simulink model "PX4_Run_Mode_R2016b"  (R2017b)
settings: Solver=FixedStepDiscrete  StartTime=0.0  StopTime=inf  FixedStep=Ts  RelTol=1e-3  EnableMultiTasking=on
InitFcn:
  | run('InitFcn_R2016b.m');
values from neighbouring files (symbols this model uses):
  A = Pixhawk_CSC.Parameter( {single([diag([1 1 1]) Ts*diag([1 1 1]); diag([0 0 0]) diag([1 1 1])]),'A'} )    [InitFcn.m]    (also in InitFcn_R2016b.m; InitFcn_R2017b_no_csc.m = single([diag([1 1 1]) Ts*diag([1 1 1]); diag([0 0 0]) diag([)
  app = Pixhawk_CSC.Parameter({single( [0.05; 0.05; 0.05]),'app'} )    [InitFcn.m]    (also in InitFcn_R2016b.m; InitFcn_R2017b_no_csc.m = single( [0.05; 0.05; 0.05]))
  B = Pixhawk_CSC.Parameter( {single([Ts^2/2*diag([1 1 1]); Ts*diag([1 1 1])]),'B'} )    [InitFcn.m]    (also in InitFcn_R2016b.m; InitFcn_R2017b_no_csc.m = single([Ts^2/2*diag([1 1 1]); Ts*diag([1 1 1])]))
  Beta = Pixhawk_CSC.Parameter({single( 0.02),'Beta'} )    [InitFcn.m]    (also in InitFcn_R2016b.m; InitFcn_R2017b_no_csc.m = single( 0.02))
  C = Pixhawk_CSC.Parameter( {single([diag([1 1 1]) 0*diag([1 1 1]); zeros(1,2) 1 zeros(1,3)]),'C'} )    [InitFcn.m]    (also in InitFcn_R2016b.m; InitFcn_R2017b_no_csc.m = single([diag([1 1 1]) 0*diag([1 1 1]); zeros(1,2) 1 zeros(1,)
  C1 = Pixhawk_CSC.Parameter({single( 1.08680),'C1'} )    [InitFcn.m]    (also in InitFcn_R2016b.m; InitFcn_R2017b_no_csc.m = single( 1.08680))
  C10 = Pixhawk_CSC.Parameter({single( 0.0000),'C10'} )    [InitFcn.m]    (also in InitFcn_R2016b.m; InitFcn_R2017b_no_csc.m = single( 0.0000))
  C11 = Pixhawk_CSC.Parameter({single(-0.2300),'C11'} )    [InitFcn.m]    (also in InitFcn_R2016b.m; InitFcn_R2017b_no_csc.m = single(-0.2300))
  C12 = Pixhawk_CSC.Parameter({single( 0.0000),'C12'} )    [InitFcn.m]    (also in InitFcn_R2016b.m; InitFcn_R2017b_no_csc.m = single( 0.0000))
  C13 = Pixhawk_CSC.Parameter({single( 0.8000),'C13'} )    [InitFcn.m]    (also in InitFcn_R2016b.m; InitFcn_R2017b_no_csc.m = single( 0.8000))
  C14 = Pixhawk_CSC.Parameter({single( 0.8000),'C14'} )    [InitFcn.m]    (also in InitFcn_R2016b.m; InitFcn_R2017b_no_csc.m = single( 0.8000))
  C15 = Pixhawk_CSC.Parameter({single( 1.73200),'C15'} )    [InitFcn.m]    (also in InitFcn_R2016b.m; InitFcn_R2017b_no_csc.m = single( 1.73200))
  C16 = Pixhawk_CSC.Parameter({single( 0.1000),'C16'} )    [InitFcn.m]    (also in InitFcn_R2016b.m; InitFcn_R2017b_no_csc.m = single( 0.1000))
  C17 = Pixhawk_CSC.Parameter({single( 0.1000),'C17'} )    [InitFcn.m]    (also in InitFcn_R2016b.m; InitFcn_R2017b_no_csc.m = single( 0.1000))
  C18 = Pixhawk_CSC.Parameter({single( 0.0500),'C18'} )    [InitFcn.m]    (also in InitFcn_R2016b.m; InitFcn_R2017b_no_csc.m = single( 0.0500))
  C19 = Pixhawk_CSC.Parameter({single( 0.6000),'C19'} )    [InitFcn.m]    (also in InitFcn_R2016b.m; InitFcn_R2017b_no_csc.m = single( 0.6000))
  C2 = Pixhawk_CSC.Parameter({single( 1.10468),'C2'} )    [InitFcn.m]    (also in InitFcn_R2016b.m; InitFcn_R2017b_no_csc.m = single( 1.10468))
  C20 = Pixhawk_CSC.Parameter({single( 0.6000),'C20'} )    [InitFcn.m]    (also in InitFcn_R2016b.m; InitFcn_R2017b_no_csc.m = single( 0.6000))
  C21 = Pixhawk_CSC.Parameter({single( 1.04558),'C21'} )    [InitFcn.m]    (also in InitFcn_R2016b.m; InitFcn_R2017b_no_csc.m = single( 1.04558))
  C22 = Pixhawk_CSC.Parameter({single( 0.0000),'C22'} )    [InitFcn.m]    (also in InitFcn_R2016b.m; InitFcn_R2017b_no_csc.m = single( 0.0000))
  C23 = Pixhawk_CSC.Parameter({single( 0.0000),'C23'} )    [InitFcn.m]    (also in InitFcn_R2016b.m; InitFcn_R2017b_no_csc.m = single( 0.0000))
  C24 = Pixhawk_CSC.Parameter({single(-11.0000),'C24'} )    [InitFcn.m]    (also in InitFcn_R2016b.m; InitFcn_R2017b_no_csc.m = single(-11.0000))
  C3 = Pixhawk_CSC.Parameter({single( 1.1980),'C3'} )    [InitFcn.m]    (also in InitFcn_R2016b.m; InitFcn_R2017b_no_csc.m = single( 1.1980))
  C4 = Pixhawk_CSC.Parameter({single( 0.0500),'C4'} )    [InitFcn.m]    (also in InitFcn_R2016b.m; InitFcn_R2017b_no_csc.m = single( 0.0500))
  C5 = Pixhawk_CSC.Parameter({single( 0.0500),'C5'} )    [InitFcn.m]    (also in InitFcn_R2016b.m; InitFcn_R2017b_no_csc.m = single( 0.0500))
  C6 = Pixhawk_CSC.Parameter({single( 0.0500),'C6'} )    [InitFcn.m]    (also in InitFcn_R2016b.m; InitFcn_R2017b_no_csc.m = single( 0.0500))
  C7 = Pixhawk_CSC.Parameter({single( 0.35937),'C7'} )    [InitFcn.m]    (also in InitFcn_R2016b.m; InitFcn_R2017b_no_csc.m = single( 0.35937))
  C8 = Pixhawk_CSC.Parameter({single( 0.36528),'C8'} )    [InitFcn.m]    (also in InitFcn_R2016b.m; InitFcn_R2017b_no_csc.m = single( 0.36528))
  C9 = Pixhawk_CSC.Parameter({single( 0.53311),'C9'} )    [InitFcn.m]    (also in InitFcn_R2016b.m; InitFcn_R2017b_no_csc.m = single( 0.53311))
  C_1 = Pixhawk_CSC.Parameter( {single([diag([1 1 1]) 0*diag([1 1 1])]),'C1'} )    [InitFcn.m]    (also in InitFcn_R2016b.m; InitFcn_R2017b_no_csc.m = single([diag([1 1 1]) 0*diag([1 1 1])]))
  CAL_ACC0_XOFFSET = Pixhawk_CSC.Parameter( {single( 0.122052  ),'CAL_ACC0_XOFFSET'} )    [InitFcn.m]    (also in InitFcn_R2016b.m; InitFcn_R2017b_no_csc.m = single( 0.122052  ))
  CAL_ACC0_XXSCALE = Pixhawk_CSC.Parameter( {single(  1.01218    ),'CAL_ACC0_XXSCALE'} )    [InitFcn.m]    (also in InitFcn_R2016b.m; InitFcn_R2017b_no_csc.m = single(  1.01218    ))
  CAL_ACC0_XYSCALE = Pixhawk_CSC.Parameter( {single( -0.00443301 ),'CAL_ACC0_XYSCALE'} )    [InitFcn.m]    (also in InitFcn_R2016b.m; InitFcn_R2017b_no_csc.m = single( -0.00443301 ))
  CAL_ACC0_XZSCALE = Pixhawk_CSC.Parameter( {single( -0.00505793 ),'CAL_ACC0_XZSCALE'} )    [InitFcn.m]    (also in InitFcn_R2016b.m; InitFcn_R2017b_no_csc.m = single( -0.00505793 ))
  CAL_ACC0_YOFFSET = Pixhawk_CSC.Parameter( {single( 0.00281205),'CAL_ACC0_YOFFSET'} )    [InitFcn.m]    (also in InitFcn_R2016b.m; InitFcn_R2017b_no_csc.m = single( 0.00281205))
  CAL_ACC0_YXSCALE = Pixhawk_CSC.Parameter( {single( -0.00443301 ),'CAL_ACC0_YXSCALE'} )    [InitFcn.m]    (also in InitFcn_R2016b.m; InitFcn_R2017b_no_csc.m = single( -0.00443301 ))
  CAL_ACC0_YYSCALE = Pixhawk_CSC.Parameter( {single(  1.00234    ),'CAL_ACC0_YYSCALE'} )    [InitFcn.m]    (also in InitFcn_R2016b.m; InitFcn_R2017b_no_csc.m = single(  1.00234    ))
  CAL_ACC0_YZSCALE = Pixhawk_CSC.Parameter( {single(  0.0160883  ),'CAL_ACC0_YZSCALE'} )    [InitFcn.m]    (also in InitFcn_R2016b.m; InitFcn_R2017b_no_csc.m = single(  0.0160883  ))
  CAL_ACC0_ZOFFSET = Pixhawk_CSC.Parameter( {single(-0.0298121 ),'CAL_ACC0_ZOFFSET'} )    [InitFcn.m]    (also in InitFcn_R2016b.m; InitFcn_R2017b_no_csc.m = single(-0.0298121 ))
  CAL_ACC0_ZXSCALE = Pixhawk_CSC.Parameter( {single( -0.00505793 ),'CAL_ACC0_ZXSCALE'} )    [InitFcn.m]    (also in InitFcn_R2016b.m; InitFcn_R2017b_no_csc.m = single( -0.00505793 ))
  CAL_ACC0_ZYSCALE = Pixhawk_CSC.Parameter( {single(  0.0160883  ),'CAL_ACC0_ZYSCALE'} )    [InitFcn.m]    (also in InitFcn_R2016b.m; InitFcn_R2017b_no_csc.m = single(  0.0160883  ))
  CAL_ACC0_ZZSCALE = Pixhawk_CSC.Parameter( {single(  0.983604   ),'CAL_ACC0_ZZSCALE'} )    [InitFcn.m]    (also in InitFcn_R2016b.m; InitFcn_R2017b_no_csc.m = single(  0.983604   ))
  CAL_BAR_OFFSET = Pixhawk_CSC.Parameter( {single( -20.8468),'CAL_BAR_OFFSET'} )    [InitFcn.m]    (also in InitFcn_R2016b.m; InitFcn_R2017b_no_csc.m = single( -20.8468))
  CAL_BAR_SCALE = Pixhawk_CSC.Parameter( {single(   1.0632),'CAL_BAR_SCALE'} )    [InitFcn.m]    (also in InitFcn_R2016b.m; InitFcn_R2017b_no_csc.m = single(   1.0632))
  CAL_BAT0_XOFFSET = Pixhawk_CSC.Parameter( {single( 0.0000),'CAL_BAT0_XOFFSET'} )    [InitFcn.m]    (also in InitFcn_R2016b.m; InitFcn_R2017b_no_csc.m = single( 0.0000))
  CAL_BAT0_XXSCALE = Pixhawk_CSC.Parameter( {single(  1.0000),'CAL_BAT0_XXSCALE'} )    [InitFcn.m]    (also in InitFcn_R2016b.m; InitFcn_R2017b_no_csc.m = single(  1.0000))
  CAL_BAT0_XYSCALE = Pixhawk_CSC.Parameter( {single(  0.0000),'CAL_BAT0_XYSCALE'} )    [InitFcn.m]    (also in InitFcn_R2016b.m; InitFcn_R2017b_no_csc.m = single(  0.0000))
  CAL_BAT0_XZSCALE = Pixhawk_CSC.Parameter( {single(  0.0000),'CAL_BAT0_XZSCALE'} )    [InitFcn.m]    (also in InitFcn_R2016b.m; InitFcn_R2017b_no_csc.m = single(  0.0000))
  CAL_BAT0_YOFFSET = Pixhawk_CSC.Parameter( {single( 0.0000),'CAL_BAT0_YOFFSET'} )    [InitFcn.m]    (also in InitFcn_R2016b.m; InitFcn_R2017b_no_csc.m = single( 0.0000))
  CAL_BAT0_YXSCALE = Pixhawk_CSC.Parameter( {single(  0.0000),'CAL_BAT0_YXSCALE'} )    [InitFcn.m]    (also in InitFcn_R2016b.m; InitFcn_R2017b_no_csc.m = single(  0.0000))
  CAL_BAT0_YYSCALE = Pixhawk_CSC.Parameter( {single(  1.0000),'CAL_BAT0_YYSCALE'} )    [InitFcn.m]    (also in InitFcn_R2016b.m; InitFcn_R2017b_no_csc.m = single(  1.0000))
  CAL_BAT0_YZSCALE = Pixhawk_CSC.Parameter( {single(  0.0000),'CAL_BAT0_YZSCALE'} )    [InitFcn.m]    (also in InitFcn_R2016b.m; InitFcn_R2017b_no_csc.m = single(  0.0000))
  CAL_BAT0_ZOFFSET = Pixhawk_CSC.Parameter( {single( 0.0000),'CAL_BAT0_ZOFFSET'} )    [InitFcn.m]    (also in InitFcn_R2016b.m; InitFcn_R2017b_no_csc.m = single( 0.0000))
  CAL_BAT0_ZXSCALE = Pixhawk_CSC.Parameter( {single(  0.0000),'CAL_BAT0_ZXSCALE'} )    [InitFcn.m]    (also in InitFcn_R2016b.m; InitFcn_R2017b_no_csc.m = single(  0.0000))
  CAL_BAT0_ZYSCALE = Pixhawk_CSC.Parameter( {single(  0.0000),'CAL_BAT0_ZYSCALE'} )    [InitFcn.m]    (also in InitFcn_R2016b.m; InitFcn_R2017b_no_csc.m = single(  0.0000))
  CAL_BAT0_ZZSCALE = Pixhawk_CSC.Parameter( {single(  1.0000),'CAL_BAT0_ZZSCALE'} )    [InitFcn.m]    (also in InitFcn_R2016b.m; InitFcn_R2017b_no_csc.m = single(  1.0000))
  CAL_GPS0_XOFFSET = Pixhawk_CSC.Parameter( {single( 0.0000),'CAL_GPS0_XOFFSET'} )    [InitFcn.m]    (also in InitFcn_R2016b.m; InitFcn_R2017b_no_csc.m = single( 0.0000))
  CAL_GPS0_XXSCALE = Pixhawk_CSC.Parameter( {single(  0.0100),'CAL_GPS0_XXSCALE'} )    [InitFcn.m]    (also in InitFcn_R2016b.m; InitFcn_R2017b_no_csc.m = single(  0.0100))
  CAL_GPS0_XYSCALE = Pixhawk_CSC.Parameter( {single(  0.0000),'CAL_GPS0_XYSCALE'} )    [InitFcn.m]    (also in InitFcn_R2016b.m; InitFcn_R2017b_no_csc.m = single(  0.0000))
  CAL_GPS0_XZSCALE = Pixhawk_CSC.Parameter( {single(  0.0000),'CAL_GPS0_XZSCALE'} )    [InitFcn.m]    (also in InitFcn_R2016b.m; InitFcn_R2017b_no_csc.m = single(  0.0000))
  CAL_GPS0_YOFFSET = Pixhawk_CSC.Parameter( {single( 0.0000),'CAL_GPS0_YOFFSET'} )    [InitFcn.m]    (also in InitFcn_R2016b.m; InitFcn_R2017b_no_csc.m = single( 0.0000))
  CAL_GPS0_YXSCALE = Pixhawk_CSC.Parameter( {single(  0.0000),'CAL_GPS0_YXSCALE'} )    [InitFcn.m]    (also in InitFcn_R2016b.m; InitFcn_R2017b_no_csc.m = single(  0.0000))
  CAL_GPS0_YYSCALE = Pixhawk_CSC.Parameter( {single(  0.0100),'CAL_GPS0_YYSCALE'} )    [InitFcn.m]    (also in InitFcn_R2016b.m; InitFcn_R2017b_no_csc.m = single(  0.0100))
  CAL_GPS0_YZSCALE = Pixhawk_CSC.Parameter( {single(  0.0000),'CAL_GPS0_YZSCALE'} )    [InitFcn.m]    (also in InitFcn_R2016b.m; InitFcn_R2017b_no_csc.m = single(  0.0000))
  CAL_GPS0_ZOFFSET = Pixhawk_CSC.Parameter( {single( 0.0000),'CAL_GPS0_ZOFFSET'} )    [InitFcn.m]    (also in InitFcn_R2016b.m; InitFcn_R2017b_no_csc.m = single( 0.0000))
  CAL_GPS0_ZXSCALE = Pixhawk_CSC.Parameter( {single(  0.0000),'CAL_GPS0_ZXSCALE'} )    [InitFcn.m]    (also in InitFcn_R2016b.m; InitFcn_R2017b_no_csc.m = single(  0.0000))
  CAL_GPS0_ZYSCALE = Pixhawk_CSC.Parameter( {single(  0.0000),'CAL_GPS0_ZYSCALE'} )    [InitFcn.m]    (also in InitFcn_R2016b.m; InitFcn_R2017b_no_csc.m = single(  0.0000))
  CAL_GPS0_ZZSCALE = Pixhawk_CSC.Parameter( {single( -0.0010),'CAL_GPS0_ZZSCALE'} )    [InitFcn.m]    (also in InitFcn_R2016b.m; InitFcn_R2017b_no_csc.m = single( -0.0010))
  CAL_GYRO0_XXSCALE = Pixhawk_CSC.Parameter( {single(0.992736),'CAL_GYRO0_XXSCALE'} )    [InitFcn.m]    (also in InitFcn_R2016b.m; InitFcn_R2017b_no_csc.m = single(0.992736))
  CAL_GYRO0_XYSCALE = Pixhawk_CSC.Parameter( {single(0.0000),'CAL_GYRO0_XYSCALE'} )    [InitFcn.m]    (also in InitFcn_R2016b.m; InitFcn_R2017b_no_csc.m = single(0.0000))
  CAL_GYRO0_XZSCALE = Pixhawk_CSC.Parameter( {single(0.0000),'CAL_GYRO0_XZSCALE'} )    [InitFcn.m]    (also in InitFcn_R2016b.m; InitFcn_R2017b_no_csc.m = single(0.0000))
  CAL_GYRO0_YXSCALE = Pixhawk_CSC.Parameter( {single(0.0000),'CAL_GYRO0_YXSCALE'} )    [InitFcn.m]    (also in InitFcn_R2016b.m; InitFcn_R2017b_no_csc.m = single(0.0000))
  CAL_GYRO0_YYSCALE = Pixhawk_CSC.Parameter( {single(1.01609),'CAL_GYRO0_YYSCALE'} )    [InitFcn.m]    (also in InitFcn_R2016b.m; InitFcn_R2017b_no_csc.m = single(1.01609))
  CAL_GYRO0_YZSCALE = Pixhawk_CSC.Parameter( {single(0.0000),'CAL_GYRO0_YZSCALE'} )    [InitFcn.m]    (also in InitFcn_R2016b.m; InitFcn_R2017b_no_csc.m = single(0.0000))
  CAL_GYRO0_ZXSCALE = Pixhawk_CSC.Parameter( {single(0.0000),'CAL_GYRO0_ZXSCALE'} )    [InitFcn.m]    (also in InitFcn_R2016b.m; InitFcn_R2017b_no_csc.m = single(0.0000))
  CAL_GYRO0_ZYSCALE = Pixhawk_CSC.Parameter( {single(0.0000),'CAL_GYRO0_ZYSCALE'} )    [InitFcn.m]    (also in InitFcn_R2016b.m; InitFcn_R2017b_no_csc.m = single(0.0000))
  CAL_GYRO0_ZZSCALE = Pixhawk_CSC.Parameter( {single(1.03003),'CAL_GYRO0_ZZSCALE'} )    [InitFcn.m]    (also in InitFcn_R2016b.m; InitFcn_R2017b_no_csc.m = single(1.03003))
  CAL_MAG0_XCURCOR = Pixhawk_CSC.Parameter( {single( 0.0017     ),'CAL_MAG0_XCURCOR'} )    [InitFcn.m]    (also in InitFcn_R2016b.m; InitFcn_R2017b_no_csc.m = single( 0.0017     ))
  CAL_MAG0_XOFFSET = Pixhawk_CSC.Parameter( {single( 0.0446372  ),'CAL_MAG0_XOFFSET'} )    [InitFcn.m]    (also in InitFcn_R2016b.m; InitFcn_R2017b_no_csc.m = single( 0.0446372  ))
  CAL_MAG0_XXSCALE = Pixhawk_CSC.Parameter( {single(  1.01563   ),'CAL_MAG0_XXSCALE'} )    [InitFcn.m]    (also in InitFcn_R2016b.m; InitFcn_R2017b_no_csc.m = single(  1.01563   ))
  CAL_MAG0_XYSCALE = Pixhawk_CSC.Parameter( {single( -0.0612061 ),'CAL_MAG0_XYSCALE'} )    [InitFcn.m]    (also in InitFcn_R2016b.m; InitFcn_R2017b_no_csc.m = single( -0.0612061 ))
  CAL_MAG0_XZSCALE = Pixhawk_CSC.Parameter( {single( -0.011532  ),'CAL_MAG0_XZSCALE'} )    [InitFcn.m]    (also in InitFcn_R2016b.m; InitFcn_R2017b_no_csc.m = single( -0.011532  ))
  CAL_MAG0_YCURCOR = Pixhawk_CSC.Parameter( {single(-0.0075     ),'CAL_MAG0_YCURCOR'} )    [InitFcn.m]    (also in InitFcn_R2016b.m; InitFcn_R2017b_no_csc.m = single(-0.0075     ))
  CAL_MAG0_YOFFSET = Pixhawk_CSC.Parameter( {single( 0.0700776  ),'CAL_MAG0_YOFFSET'} )    [InitFcn.m]    (also in InitFcn_R2016b.m; InitFcn_R2017b_no_csc.m = single( 0.0700776  ))
  CAL_MAG0_YXSCALE = Pixhawk_CSC.Parameter( {single( -0.0612061 ),'CAL_MAG0_YXSCALE'} )    [InitFcn.m]    (also in InitFcn_R2016b.m; InitFcn_R2017b_no_csc.m = single( -0.0612061 ))
  CAL_MAG0_YYSCALE = Pixhawk_CSC.Parameter( {single(  1.00593   ),'CAL_MAG0_YYSCALE'} )    [InitFcn.m]    (also in InitFcn_R2016b.m; InitFcn_R2017b_no_csc.m = single(  1.00593   ))
  CAL_MAG0_YZSCALE = Pixhawk_CSC.Parameter( {single(  0.0144582 ),'CAL_MAG0_YZSCALE'} )    [InitFcn.m]    (also in InitFcn_R2016b.m; InitFcn_R2017b_no_csc.m = single(  0.0144582 ))
  CAL_MAG0_ZCURCOR = Pixhawk_CSC.Parameter( {single(-0.0080     ),'CAL_MAG0_ZCURCOR'} )    [InitFcn.m]    (also in InitFcn_R2016b.m; InitFcn_R2017b_no_csc.m = single(-0.0080     ))
  CAL_MAG0_ZOFFSET = Pixhawk_CSC.Parameter( {single( 0.00201742 ),'CAL_MAG0_ZOFFSET'} )    [InitFcn.m]    (also in InitFcn_R2016b.m; InitFcn_R2017b_no_csc.m = single( 0.00201742 ))
  CAL_MAG0_ZXSCALE = Pixhawk_CSC.Parameter( {single( -0.011532  ),'CAL_MAG0_ZXSCALE'} )    [InitFcn.m]    (also in InitFcn_R2016b.m; InitFcn_R2017b_no_csc.m = single( -0.011532  ))
  CAL_MAG0_ZYSCALE = Pixhawk_CSC.Parameter( {single(  0.0144582 ),'CAL_MAG0_ZYSCALE'} )    [InitFcn.m]    (also in InitFcn_R2016b.m; InitFcn_R2017b_no_csc.m = single(  0.0144582 ))
  CAL_MAG0_ZZSCALE = Pixhawk_CSC.Parameter( {single(  0.986813  ),'CAL_MAG0_ZZSCALE'} )    [InitFcn.m]    (also in InitFcn_R2016b.m; InitFcn_R2017b_no_csc.m = single(  0.986813  ))
  CAL_SONAR_OFFSET = Pixhawk_CSC.Parameter( {single( -6.8730),'CAL_SONAR_OFFSET'} )    [InitFcn.m]    (also in InitFcn_R2016b.m; InitFcn_R2017b_no_csc.m = single( -6.8730))
  CAL_SONAR_SCALE = Pixhawk_CSC.Parameter( {single(-438.1875),'CAL_SONAR_SCALE'} )    [InitFcn.m]    (also in InitFcn_R2016b.m; InitFcn_R2017b_no_csc.m = single(-438.1875))
  COM_RATE = double(10)    [InitFcn.m]    (also in InitFcn_R2016b.m; InitFcn_R2017b_no_csc.m)
  D = Pixhawk_CSC.Parameter( {single(zeros(size(C.Value,1), size(B.Value,2))),'D'} )    [InitFcn.m]    (also in InitFcn_R2016b.m; InitFcn_R2017b_no_csc.m = single(zeros(size(C,1), size(B,2))))
  Dip0 = Pixhawk_CSC.Parameter({single( 1.2),'Dip0'} )    [InitFcn.m]    (also in InitFcn_R2016b.m; InitFcn_R2017b_no_csc.m = single( 1.2))
  I = Pixhawk_CSC.Parameter( {single(eye(size(Q.Value))),'I'} )    [InitFcn.m]    (also in InitFcn_R2016b.m; InitFcn_R2017b_no_csc.m = single(eye(size(Q))))
  Jxx = Pixhawk_CSC.Parameter( {single(J(1,1)),'Jxx'} )    [InitFcn.m]    (also in InitFcn_R2016b.m; InitFcn_R2017b_no_csc.m = single(J(1,1)))
  Jyy = Pixhawk_CSC.Parameter( {single(J(2,2)),'Jyy'} )    [InitFcn.m]    (also in InitFcn_R2016b.m; InitFcn_R2017b_no_csc.m = single(J(2,2)))
  Jzz = Pixhawk_CSC.Parameter( {single(J(3,3)),'Jzz'} )    [InitFcn.m]    (also in InitFcn_R2016b.m; InitFcn_R2017b_no_csc.m = single(J(3,3)))
  Kapp = Pixhawk_CSC.Parameter({single( 1.2),'Kapp'} )    [InitFcn.m]    (also in InitFcn_R2016b.m; InitFcn_R2017b_no_csc.m = single( 1.2))
  Kx = Pixhawk_CSC.Parameter({single( Kx),'Kx'} )    [InitFcn.m]    (also in InitFcn_R2016b.m = Pixhawk_CSC.Parameter({single( [0.60 0.9]),'Kx'} ); InitFcn_R2017b_no_csc.m = single( [0.60 0.9]))
  Ky = Pixhawk_CSC.Parameter({single( Ky),'Ky'} )    [InitFcn.m]    (also in InitFcn_R2016b.m = Pixhawk_CSC.Parameter({single( [0.4 0.9]),'Ky'} ); InitFcn_R2017b_no_csc.m = single( [0.4 0.9]))
  LPF_REF_DEN = Pixhawk_CSC.Parameter( {single([1.0000 -0.8187]),'LPF_REF_DEN'} )    [InitFcn.m]    (also in InitFcn_R2016b.m; InitFcn_R2017b_no_csc.m = single([1.0000 -0.8187]))
  LPF_REF_NUM = Pixhawk_CSC.Parameter( {single([0.0000  0.1813]),'LPF_REF_NUM'} )    [InitFcn.m]    (also in InitFcn_R2016b.m; InitFcn_R2017b_no_csc.m = single([0.0000  0.1813]))
  m0 = Pixhawk_CSC.Parameter({single( 0.452857),'m0'} )    [InitFcn.m]    (also in InitFcn_R2016b.m; InitFcn_R2017b_no_csc.m = single( 0.452857))
  mn = [0.01; 0.01; 0.01; 0.01]    [InitFcn.m]    (also in InitFcn_R2016b.m; InitFcn_R2017b_no_csc.m)
  MOV_AVG_WINDOW = Pixhawk_CSC.Parameter( {single(100),'MOV_AVG_WINDOW'} )    [InitFcn.m]    (also in InitFcn_R2016b.m; InitFcn_R2017b_no_csc.m = single(100))
  Ox0 = Pixhawk_CSC.Parameter({single(O_x0),'Ox0'} )    [InitFcn.m]    (also in InitFcn_R2016b.m; InitFcn_R2017b_no_csc.m = single(O_x0))
  Oxa = Pixhawk_CSC.Parameter({single(O_x.a),'Oxa'} )    [InitFcn.m]    (also in InitFcn_R2016b.m; InitFcn_R2017b_no_csc.m = single(O_x.a))
  Oxb = Pixhawk_CSC.Parameter({single(O_x.b),'Oxb'} )    [InitFcn.m]    (also in InitFcn_R2016b.m; InitFcn_R2017b_no_csc.m = single(O_x.b))
  Oxc = Pixhawk_CSC.Parameter({single(O_x.c),'Oxc'} )    [InitFcn.m]    (also in InitFcn_R2016b.m; InitFcn_R2017b_no_csc.m = single(O_x.c))
  Oxd = Pixhawk_CSC.Parameter({single(O_x.d),'Oxd'} )    [InitFcn.m]    (also in InitFcn_R2016b.m; InitFcn_R2017b_no_csc.m = single(O_x.d))
  Oy0 = Pixhawk_CSC.Parameter({single(O_y0),'Oy0'} )    [InitFcn.m]    (also in InitFcn_R2016b.m; InitFcn_R2017b_no_csc.m = single(O_y0))
  Oya = Pixhawk_CSC.Parameter({single(O_y.a),'Oya'} )    [InitFcn.m]    (also in InitFcn_R2016b.m; InitFcn_R2017b_no_csc.m = single(O_y.a))
  Oyb = Pixhawk_CSC.Parameter({single(O_y.b),'Oyb'} )    [InitFcn.m]    (also in InitFcn_R2016b.m; InitFcn_R2017b_no_csc.m = single(O_y.b))
  Oyc = Pixhawk_CSC.Parameter({single(O_y.c),'Oyc'} )    [InitFcn.m]    (also in InitFcn_R2016b.m; InitFcn_R2017b_no_csc.m = single(O_y.c))
  Oyd = Pixhawk_CSC.Parameter({single(O_y.d),'Oyd'} )    [InitFcn.m]    (also in InitFcn_R2016b.m; InitFcn_R2017b_no_csc.m = single(O_y.d))
  Oz0 = Pixhawk_CSC.Parameter({single(O_z0),'Oz0'} )    [InitFcn.m]    (also in InitFcn_R2016b.m; InitFcn_R2017b_no_csc.m = single(O_z0))
  ... (+53 more)
undefined symbols (not defined in the file or in its folder): AccX, AccY, AccZ, Altitude, ax, ay, az, Current, FILTER_N, GPS_TS, GyroX, GyroY, GyroZ, Latitude, Longitude, M1_PWM, M2_PWM, M3_PWM, M4_PWM, MagX, MagY, MagZ, mAH, MOTOR, phi, Position_TS, psi, PX4_TUNE_ENUM, RGBLED_COLOR_ENUM, RGBLED_MODE_ENUM, S_AccX, S_AccY, S_AccZ, S_Altitude, S_Baro, S_Current, S_GyroX, S_GyroY, S_GyroZ, S_Latitude, S_Longitude, S_MagX, S_MagY, S_MagZ, S_mAH, S_N_Sat, S_Voltage, T_PITCH, T_ROLL, T_THROTTLE, theta, v, Voltage, w, wx, wxd, wy, wyd, wz ... (+4)
libraries: simulink x31, pixhawk_slib_sensors_actuators x7, pixhawk_slib_ADC_serial x5, pixhawk_slib_misc_utils x3, etargetslib x2
(part 7 of 7)

== matlab function PX4_Run_Mode_R2016b/RC_FILTER/Scale_Roll_RC1 ==
  data: RC_Roll input; T_Y output; RC1_MAX parameter; RC1_MIN parameter; RC1_TRIM parameter; RC1_DB parameter; Y_MAX parameter
function T_Y = Scale_Roll_RC(RC_Roll, RC1_MAX, RC1_MIN, RC1_TRIM, RC1_DB, Y_MAX)

%% Initialize variable
T_Y = single(0);
RC_Roll = single(RC_Roll);

%% Transform RC channel input to desired values
% RC channel 1 [984    , 1499    , 2006]
%              [RC1_MIN, RC1_TRIM, RC1_MAX]

% Test if RC was once connected, or still is connected
T_Y = RC_Roll - RC1_TRIM;
if(T_Y < -RC1_DB)
    T_Y = T_Y/(RC1_TRIM - RC1_MIN);
elseif(T_Y > RC1_DB)
    T_Y = T_Y/(RC1_MAX - RC1_TRIM);
else
    T_Y = single(0);
end


%% Limit output to [-1, 1]
if(RC_Roll == 0)
    T_Y = single(0);
else
    if(T_Y > 1)
        T_Y = single(1);
    elseif(T_Y < -1)
        T_Y = single(-1);
    end
end

%% Scale output to [MIN MAX] Roll value
T_Y = T_Y * Y_MAX;
if(T_Y > Y_MAX)
    T_Y = single(Y_MAX);
elseif(T_Y < -Y_MAX)
    T_Y = single(-Y_MAX);
end

== matlab function PX4_Run_Mode_R2016b/SENSOR_FILTER/Fixed Bias removal and scaling/Parameter Bus Creation/Initial State Bias/Initiate_State_Bias ==
  data: BIAS_STATE output
function BIAS_STATE = INIT_STATE_BIAS

BIAS_STATE = single([0; 0; 0;... 
                     0; 0; 0;... 
                     0; 0; 0;... 
                     0; 0; 0;... 
                     0; 0; 0;... 
                     0; 0; 0]);

== matlab function PX4_Run_Mode_R2016b/SENSOR_FILTER/Fixed Bias removal and scaling/GPS Calibration/GYRO_BIAS ==
  data: GPS_IN input; RESET input; CONFIG_CMD input; MOV_AVG_WINDOW parameter; BGPS output
function BGPS = GPSBias(GPS_IN, RESET, CONFIG_CMD, MOV_AVG_WINDOW)

GPSx = GPS_IN(1);
GPSy = GPS_IN(2);
GPSz = GPS_IN(3);

%% Initiate BIAS memory
persistent BIAS;
if(isempty(BIAS) || RESET)
    BIAS = single([0; 0; 0]);
end

BGPS = single([0; 0; 0]);

%% If Pre-Armed, average input
if(CONFIG_CMD)
    BIAS(1) = BIAS(1) + GPSx/MOV_AVG_WINDOW;
    BIAS(2) = BIAS(2) + GPSy/MOV_AVG_WINDOW;
    BIAS(3) = BIAS(3) + GPSz/MOV_AVG_WINDOW;
end

%% Outputs
BGPS = BIAS;

== matlab function PX4_Run_Mode_R2016b/SENSOR_FILTER/SensorData2States/Rotational State Estimation/AHRS ==
  data: M input; Reset input; A input; q output; G input; Ts parameter; app parameter; Kapp parameter; thg parameter; m0 parameter; Dip0 parameter; thdip parameter; Beta parameter
function q = MadgwickAHRS(M, Reset, A, G, Ts, app, Kapp, thg, m0, Dip0, thdip, Beta)
% A ==> Accelerometer data in x, y, z direction
% M ==> Magnetometer data in x, y, z direction
% G ==> Gyroscope data in x, y, z direction
%% Parameters
% app = [1; 1; 1];        % Maximum expected acceleration during stationary state (peak - peak)
% Kapp = 1.2;             % Stationary state detection accelerometer detection
% thg = [1; 1; 1];        % Maximum expected gyroscope during stationary state (bound)
% m0 = 1;                 % Expected Magnetometer magnitude
% Dip0 = 0.6;             % Expected Dip angle under undisturbed operation
% thdip = 0.5;            % Scaling dip error
% Beta = 0.1;             % Gradient Descent Step size

g = [0; 0; 1];          % Gravity vector
% Ts = 1/400;             % Sampling time


%% Initialization
tha = Kapp * app;

% Previous measured accelerations
persistent A_old        
if(isempty(A_old))
    A_old = single(zeros(3,1));
end

% Previous estimated quaternions
persistent q_old        
if(isempty(q_old))
    q_old = single([1, zeros(1,3)]);
end

% Rotation Matrix
R = zeros(3,3);
ab = zeros(1,4);
Lambda_1 = 0;
Lambda_2 = 0;
Lambda = 0;

%% Estimate MIMU quaternions
q_mimu = q_old;

% Normalise accelerometer measurement
Acc = A / norm(A);  % normalise magnitude

% Normalise magnetometer measurement
Mag = M / norm(M);  % normalise magnitude

% Reference direction of Earth's magnetic field
q_mimuConj = [q_mimu(:,1) -q_mimu(:,2) -q_mimu(:,3) -q_mimu(:,4)];
q_Mag = [0 Mag'];

a = q_Mag; b = q_mimuConj;
ab(:,1) = a(:,1).*b(:,1)-a(:,2).*b(:,2)-a(:,3).*b(:,3)-a(:,4).*b(:,4);
ab(:,2) = a(:,1).*b(:,2)+a(:,2).*b(:,1)+a(:,3).*b(:,4)-a(:,4).*b(:,3);
ab(:,3) = a(:,1).*b(:,3)-a(:,2).*b(:,4)+a(:,3).*b(:,1)+a(:,4).*b(:,2);
ab(:,4) = a(:,1).*b(:,4)+a(:,2).*b(:,3)-a(:,3).*b(:,2)+a(:,4).*b(:,1);

a = q_mimu; b = ab;
ab(:,1) = a(:,1).*b(:,1)-a(:,2).*b(:,2)-a(:,3).*b(:,3)-a(:,4).*b(:,4);
ab(:,2) = a(:,1).*b(:,2)+a(:,2).*b(:,1)+a(:,3).*b(:,4)-a(:,4).*b(:,3);
ab(:,3) = a(:,1).*b(:,3)-a(:,2).*b(:,4)+a(:,3).*b(:,1)+a(:,4).*b(:,2);
ab(:,4) = a(:,1).*b(:,4)+a(:,2).*b(:,3)-a(:,3).*b(:,2)+a(:,4).*b(:,1);

h = ab;
b = [0 norm([h(2) h(3)]) 0 h(4)];

% Gradient decent algorithm corrective step
 F_mimu = [2*(q_mimu(2)*q_mimu(4) - q_mimu(1)*q_mimu(3)) - Acc(1)
      2*(q_mimu(1)*q_mimu(2) + q_mimu(3)*q_mimu(4)) - Acc(2)
      2*(0.5 - q_mimu(2)^2 - q_mimu(3)^2) - Acc(3)
      2*b(2)*(0.5 - q_mimu(3)^2 - q_mimu(4)^2) + 2*b(4)*(q_mimu(2)*q_mimu(4) - q_mimu(1)*q_mimu(3)) - Mag(1)
      2*b(2)*(q_mimu(2)*q_mimu(3) - q_mimu(1)*q_mimu(4)) + 2*b(4)*(q_mimu(1)*q_mimu(2) + q_mimu(3)*q_mimu(4)) - Mag(2)
      2*b(2)*(q_mimu(1)*q_mimu(3) + q_mimu(2)*q_mimu(4)) + 2*b(4)*(0.5 - q_mimu(2)^2 - q_mimu(3)^2) - Mag(3)];
  
J_mimu = [-2*q_mimu(3),                          2*q_mimu(4),                        -2*q_mimu(1),                       2*q_mimu(2)
     2*q_mimu(2),                           2*q_mimu(1),                        2*q_mimu(4),                        2*q_mimu(3)
     0,                                     -4*q_mimu(2),                       -4*q_mimu(3),                       0
     -2*b(4)*q_mimu(3),                     2*b(4)*q_mimu(4),                   -4*b(2)*q_mimu(3)-2*b(4)*q_mimu(1), -4*b(2)*q_mimu(4)+2*b(4)*q_mimu(2)
     -2*b(2)*q_mimu(4)+2*b(4)*q_mimu(2),    2*b(2)*q_mimu(3)+2*b(4)*q_mimu(1),  2*b(2)*q_mimu(2)+2*b(4)*q_mimu(4),  -2*b(2)*q_mimu(1)+2*b(4)*q_mimu(3)
     2*b(2)*q_mimu(3),                      2*b(2)*q_mimu(4)-4*b(4)*q_mimu(2),  2*b(2)*q_mimu(1)-4*b(4)*q_mimu(3),  2*b(2)*q_mimu(2)];
step_mimu = (J_mimu'*F_mimu);
step_mimu = step_mimu/norm(step_mimu);     % normalise step magnitude

% Compute rate of change of quaternion
Gyro = [0 G(1) G(2) G(3)];
a = q_mimu; b = Gyro;
ab(:,1) = a(:,1).*b(:,1)-a(:,2).*b(:,2)-a(:,3).*b(:,3)-a(:,4).*b(:,4);
ab(:,2) = a(:,1).*b(:,2)+a(:,2).*b(:,1)+a(:,3).*b(:,4)-a(:,4).*b(:,3);
ab(:,3) = a(:,1).*b(:,3)-a(:,2).*b(:,4)+a(:,3).*b(:,1)+a(:,4).*b(:,2);
ab(:,4) = a(:,1).*b(:,4)+a(:,2).*b(:,3)-a(:,3).*b(:,2)+a(:,4).*b(:,1);
qDot_mimu = 0.5 * ab - Beta * step_mimu';

% Integrate to yield quaternion
q_mimu = q_mimu + qDot_mimu * Ts;
q_mimu = q_mimu / norm(q_mimu);     % normalise quaternion

%% Estimate IMU quaternions
q_imu = q_old;

% Normalise accelerometer measurement
Acc = A / norm(A);  % normalise magnitude

% Gradient decent algorithm corrective step
 F_imu = [2*(q_imu(2)*q_imu(4) - q_imu(1)*q_imu(3)) - Acc(1)
      2*(q_imu(1)*q_imu(2) + q_imu(3)*q_imu(4)) - Acc(2)
      2*(0.5 - q_imu(2)^2 - q_imu(3)^2) - Acc(3)];
J_imu = [-2*q_imu(3),  2*q_imu(4),     -2*q_imu(1),    2*q_imu(2)
          2*q_imu(2),   2*q_imu(1),     2*q_imu(4),     2*q_imu(3)
          0,            -4*q_imu(2),    -4*q_imu(3),    0];
step_imu = (J_imu'*F_imu);
step_imu = step_imu/norm(step_imu);     % normalise step magnitude

% Compute rate of change of quaternion
Gyro = [0 G(1) G(2) G(3)];
a = q_imu; b = Gyro;
ab(:,1) = a(:,1).*b(:,1)-a(:,2).*b(:,2)-a(:,3).*b(:,3)-a(:,4).*b(:,4);
ab(:,2) = a(:,1).*b(:,2)+a(:,2).*b(:,1)+a(:,3).*b(:,4)-a(:,4).*b(:,3);
ab(:,3) = a(:,1).*b(:,3)-a(:,2).*b(:,4)+a(:,3).*b(:,1)+a(:,4).*b(:,2);
ab(:,4) = a(:,1).*b(:,4)+a(:,2).*b(:,3)-a(:,3).*b(:,2)+a(:,4).*b(:,1);

qDot_imu = 0.5 * ab - Beta * step_imu';

% Integrate to yield quaternion
q_imu = q_imu + qDot_imu * Ts;
q_imu = q_imu / norm(q_imu);     % normalise quaternion


%% Stationary State Detection
if( (abs(A(1) - A_old(1)) < tha(1)) & (abs(A(2) - A_old(2)) < tha(2)) & (abs(A(3) - A_old(3)) < tha(3)) & (abs(G(1)) < thg(1)) & (abs(G(2)) < thg(2)) & (abs(G(3)) < thg(3)) )
    % Stationary state detected
    q = q_old;
else
    % Non-stationary state 
    R(1,1,:) = 2.*q_imu(:,1).^2-1+2.*q_imu(:,2).^2;
    R(1,2,:) = 2.*(q_imu(:,2).*q_imu(:,3)+q_imu(:,1).*q_imu(:,4));
    R(1,3,:) = 2.*(q_imu(:,2).*q_imu(:,4)-q_imu(:,1).*q_imu(:,3));
    R(2,1,:) = 2.*(q_imu(:,2).*q_imu(:,3)-q_imu(:,1).*q_imu(:,4));
    R(2,2,:) = 2.*q_imu(:,1).^2-1+2.*q_imu(:,3).^2;
    R(2,3,:) = 2.*(q_imu(:,3).*q_imu(:,4)+q_imu(:,1).*q_imu(:,2));
    R(3,1,:) = 2.*(q_imu(:,2).*q_imu(:,4)+q_imu(:,1).*q_imu(:,3));
    R(3,2,:) = 2.*(q_imu(:,3).*q_imu(:,4)-q_imu(:,1).*q_imu(:,2));
    R(3,3,:) = 2.*q_imu(:,1).^2-1+2.*q_imu(:,4).^2;
    
    H = R * M;
    
    % evaluate Magnetic Disturbance Severity
    Magnitude = sqrt(sum(M.^2)) - m0;
    Dip = (pi/2 - acos( dot(H,g)/(sqrt(dot(H,H))*sqrt(dot(g,g))) ));
    
    % Calculate Lambda's, which relates to thrustworthiness of magnetometer
    Lambda_1 = abs(Magnitude)/m0;
    if(Lambda_1 > 1), Lambda_1 = single(1); end
    
    Lambda_2 = abs(Dip - Dip0)/thdip;
    if(Lambda_2 > 1), Lambda_2 = single(1); end
    
    Lambda = (Lambda_1 + Lambda_2)/2;
    
    q = Lambda * q_imu + (1 - Lambda) * q_mimu;
end

%% Reset command given
if(Reset)
    q_old = single([1, zeros(1,3)]);
    q = single([1, zeros(1,3)]);
end

%% Save values for next iteration
A_old = A;
q_old = q;

== matlab function PX4_Run_Mode_R2016b/CONTROLLER/Ramp/Ramp1 ==
  data: Clock input; RAMP_OUT output; Reset input
function RAMP_OUT = FeedforwardRamp( Clock, Reset)

Ramp = single(0);

tstart = 1;
tend = 2;

persistent ClockZero;
if(isempty(ClockZero) || Reset)
    ClockZero = single(Clock);
end

t = single(Clock - ClockZero);

if( t > tend)
    Ramp = single(1);
elseif(t < tstart || Reset)
    Ramp = single(0);
else
    Ramp = single(t - tstart);
end

RAMP_OUT = Ramp;

== matlab function PX4_Run_Mode_R2016b/SENSOR_FILTER/Fixed Bias removal and scaling/Sonar Calibration/MATLAB Function ==
  data: Sonar_In input; Sonar_Out output; CAL_SONAR_SCALE parameter; CAL_SONAR_OFFSET parameter
function Sonar_Out = Sonar_Correction(Sonar_In, CAL_SONAR_SCALE, CAL_SONAR_OFFSET)

Sonar_Out = single(1/CAL_SONAR_SCALE*(Sonar_In - CAL_SONAR_OFFSET));

== matlab function PX4_Run_Mode_R2016b/SENSOR_FILTER/SensorData2States/Rotational State Estimation/MATLAB Function3 ==
  data: RESET input; MAG_OUT output; CONFIG_CMD input; MAG_IN input; MOV_AVG_WINDOW parameter
function MAG_OUT  = RotateMagData(RESET, CONFIG_CMD, MAG_IN, MOV_AVG_WINDOW)

%% Initiate Psi Memory
persistent PSI;
if(isempty(PSI) || RESET)
    PSI = single(0);
end

%% If Pre-Armed, average psi
if(CONFIG_CMD)
    PSI = PSI + (-atan2(MAG_IN(2), MAG_IN(1)))/MOV_AVG_WINDOW;
end

%% Remove psi from input
Rz = [cos(PSI) -sin(PSI) 0; sin(PSI) cos(PSI) 0; 0 0 1];
MAG_OUT = Rz * MAG_IN;

== matlab function PX4_Run_Mode_R2016b/CONTROLLER/Inner Control Loop/Roll Control/MATLAB Function ==
  data: Reset input; u input; y output; Ts parameter; C4 parameter
function y = Integrator(Reset, u, Ts, C4)

%% Initiate previous values
persistent u_old
if(isempty(u_old))
    u_old = single(0);
end

%% If unarmed, reset integrator
if(Reset)
    u_old = single(0);
end

u_old = u_old + single(Ts)*u*C4;

y = single(0);

== matlab function PX4_Run_Mode_R2016b/CONTROLLER/Inner Control Loop/Pitch Control/MATLAB Function ==
  data: Reset input; u input; y output; Ts parameter; C5 parameter
function y = Integrator(Reset, u, Ts, C5)

%% Initiate previous values
persistent u_old
if(isempty(u_old))
    u_old = single(0);
end

%% If unarmed, reset integrator
if(Reset)
    u_old = single(0);
end


u_old = u_old + single(Ts)*u*C5;
y = single(0);

== matlab function PX4_Run_Mode_R2016b/Communication System/Incomming Communication/MATLAB Function ==
  data: u input uint8; y output uint8
function y = FindStart(u)

ReceiveBytes = 13*4;
persistent y_old

if(isempty(y_old))
    y_old = uint8(zeros(ReceiveBytes,1));
end
y = y_old;

%% Find the line '$Drone,'
U = [u; u];
Ind = zeros(2,1);
l = 1;
crc1 = uint8(0);
crc2 = uint8(0);
for i = 1:length(U)-6
    if(U(i) == uint8('$'))
        if(U(i+1) == uint8('D'))
            if(U(i+2) == uint8('r'))
                if(U(i+3) == uint8('o'))
                    if(U(i+4) == uint8('n'))
                        if(U(i+5) == uint8('e'))
                            if(U(i+6) == uint8(','))
                                if(l<=2)
                                    Ind(l) = i;
                                    l = l + 1;
                                end
                            end
                        end
                    end
                end
            end
        end
    end
end

if(l >= 2)
    Ind(1) = Ind(1) + 7;
    Ind(2) = Ind(2) - 3;
    
    if((Ind(2) - Ind(1)) == (ReceiveBytes-1))
        crc1 = U(Ind(2)+2);
        crc2 = U(Ind(1));
        
        for i = Ind(1)+1:Ind(2)
            crc2 = bitxor(crc2, U(i));
        end
        
        if(crc1 == crc2)
%             y(1:ReceiveBytes) = U(Ind(1):Ind(1) + 7);
            % Receivebytes - 1
            y(1:ReceiveBytes) = U(Ind(1):Ind(1) + 51);
            y_old = y;
        else
            y = y_old;
        end
    end
end

== matlab function PX4_Run_Mode_R2016b/Communication System/Outgoining Communication/TrainStart ==
  data: u input uint8; y output uint8
function y = Start(u)

crc = uint8(0);
crc = u(1);
for i = 2:length(u)
    crc = bitxor(crc, u(i));
end

y = [uint8('$Drone,')'; u; uint8('*'); crc];

== matlab function PX4_Run_Mode_R2016b/SENSOR_FILTER/SensorData2States/Rotational State Estimation/MATLAB Function ==
  data: q input; phi output; theta output; psi output
function [phi, theta, psi] = quatern2TaitBryant(q)
%QUATERN2TAITBRYANT Converts a quaternion orientation to ZYX Tait Bryant angles
%
%   q = quatern2TaitBruant(q)
%
%   Converts a quaternion orientation to ZYX Tait Bryant angles where phi is a
%   rotation around X, theta around Y and psi around Z.
%
%   For more information see:
%   http://www.x-io.co.uk/node/8#quaternions
%
%	Date          Author          Notes
%	27/09/2011    SOH Madgwick    Initial release
%% Initialize variables
persistent phi_old theta_old psi_old
if(isempty(phi_old))
    phi_old = 0;
end

if(isempty(theta_old))
    theta_old = 0;
end

if(isempty(psi_old))
    psi_old = 0;
end

R = zeros(3,3);
qConj = [q(:,1) -q(:,2) -q(:,3) -q(:,4)];

%% Obtain Taint Bryant angles from quaternion
R(1,1,:) = 2.*qConj(:,1).^2-1+2.*qConj(:,2).^2;
R(2,1,:) = 2.*(qConj(:,2).*qConj(:,3)-qConj(:,1).*qConj(:,4));
R(3,1,:) = 2.*(qConj(:,2).*qConj(:,4)+qConj(:,1).*qConj(:,3));
R(3,2,:) = 2.*(qConj(:,3).*qConj(:,4)-qConj(:,1).*qConj(:,2));
R(3,3,:) = 2.*qConj(:,1).^2-1+2.*qConj(:,4).^2;

phi = atan2(R(3,2,:), R(3,3,:) );
theta = -atan(R(3,1,:) ./ sqrt(1-R(3,1,:).^2) );
psi = atan2(R(2,1,:), R(1,1,:) );

%% Unwrap angles
% Unwrap phi
if( abs(phi - phi_old) > pi )
    phi = phi - round((phi - phi_old)/pi) * pi;
end

% Unwrap theta
if( abs(theta - theta_old) > pi )
    phi = theta - round((theta - theta_old)/pi) * pi;
end

% Unwrap psi
if( abs(psi - psi_old) > pi )
    psi = psi - round((psi - psi_old)/pi) * pi;
end
    
%% Save angles for next iteration
phi_old = phi;
theta_old = theta;
psi_old = psi;

== matlab function PX4_Run_Mode_R2016b/CONTROLLER/Inner Control Loop/Yaw Control/MATLAB Function ==
  data: Reset input; e input; Ts parameter; eI output; C6 parameter
function eI = Integrator(Reset, e, Ts, C6)

persistent eI_old

if(isempty(eI_old))
    eI_old = single(0);
end

eI = eI_old + C6*e*Ts;
if(abs(eI) > 2)
    eI = sign(eI)*2;
end
eI_old = eI;

if(Reset)
    eI = single(0);
    eI_old = single(0);
end

== matlab function PX4_Run_Mode_R2016b/Communication System/Set Online Control Gains/MATLAB Function1 ==
  data: Arm input; Data_In input; Data_Out output
function Data_Out = Memory(Arm, Data_In)

%% Initiate Memory
persistent Data_Old
if(isempty(Data_Old))
    Data_Old = single([0; 0; 0;...
                       0; 0; 0;...
                       0; 0; 0;...
                       0; 0; 0;...
                       0; 0; 0;...
                       0; 0; 0;...
                       0; 0; 0;...
                       0; 0; 0]);
end
% Data_Out = zeros(size(Data_Old));

%% If drone is not armed, let the values change and saturate them
if(~Arm)
    Data_Old = Data_In;
    %% Limit Angle Gains    [1 2 3]
    for i = 1:3
        % Limit P-gains
        j = i;
        if(Data_Old(j) > 1)
            Data_Old(j) = 1;
        elseif(Data_Old(j) < 0)
            Data_Old(j) = 0;
        end        

        % Limit I-gains
        j = i+3;
        if(Data_Old(j) > 1)
            Data_Old(j) = 1;
        elseif(Data_Old(j) < 0)
            Data_Old(j) = 0;
        end
        
        % Limit D-gains
        j = i+6;
        if(Data_Old(j) > 1)
            Data_Old(j) = 1;
        elseif(Data_Old(j) < 0)
            Data_Old(j) = 0;
        end
        
        % Limit FeedForward
        j = i+9;
        if(Data_Old(j) > 1)
            Data_Old(j) = 1;
        elseif(Data_Old(j) < -1)
            Data_Old(j) = -1;
        end 
    end
    
    %% Limit Position Gains     [13 14 15]
    for i = 13:15
        % Limit P-gains
        j = i;
        if(Data_Old(j) > 5)
            Data_Old(j) = 5;
        elseif(Data_Old(j) < 0)
            Data_Old(j) = 0;
        end        

        % Limit I-gains
        j = i+3;
        if(Data_Old(j) > 1)
            Data_Old(j) = 1;
        elseif(Data_Old(j) < 0)
            Data_Old(j) = 0;
        end
        
        % Limit D-gains
        j = i+6;
        if(Data_Old(j) > 5)
            Data_Old(j) = 5;
        elseif(Data_Old(j) < 0)
            Data_Old(j) = 0;
        end
        
        % Limit FeedForward
        j = i+9;
        if(Data_Old(j) > 20)
            Data_Old(j) = 20;
        elseif(Data_Old(j) < -20)
            Data_Old(j) = -20;
        end 
    end
end

Data_Out = Data_Old;

== matlab function PX4_Run_Mode_R2016b/CONTROLLER/Outer Control Loop/Flight_Mode_Selector ==
  data: T_PITCH_OUT output; T_PITCH_IN input; T_ROLL_IN input; T_THROTTLE_IN input; U_X input; U_Y input; U_Z input; MANUAL_FLIGHT input; SEMI_AUTO_FLIGHT input; AUTO_FLIGHT input; T_ROLL_OUT output; T_THROTTLE_OUT output; psi input
function [T_PITCH_OUT, T_ROLL_OUT, T_THROTTLE_OUT] = FlightModeSelector(T_PITCH_IN, T_ROLL_IN, T_THROTTLE_IN, U_X, U_Y, U_Z, MANUAL_FLIGHT, SEMI_AUTO_FLIGHT, AUTO_FLIGHT, psi)

%% Initialize
T_PITCH_OUT     = single(0);
T_ROLL_OUT      = single(0);
T_THROTTLE_OUT  = single(0);

% World 2 Body rotations
Rz = [ cos(psi)  sin(psi) 0;...
      -sin(psi)  cos(psi) 0;...
       0         0        1];

%% Manual Flight Mode
% angles and thrust are controlled
if(MANUAL_FLIGHT)
    T_PITCH_OUT     = T_PITCH_IN;
    T_ROLL_OUT      = T_ROLL_IN;
    T_THROTTLE_OUT  = T_THROTTLE_IN;
end

%% Semi Auto Flight Mode
% angles and height are controlled
if(SEMI_AUTO_FLIGHT)
    T_PITCH_OUT     = T_PITCH_IN;
    T_ROLL_OUT      = T_ROLL_IN;
    T_THROTTLE_OUT  = U_Z;
end

%% Auto Flight Mode
% positions and height are controlled
% if(AUTO_FLIGHT)
%     T_THROTTLE_OUT  = -sqrt(U_X^2 + U_Y^2 + U_Z^2);
%     Urot            = Rz*[-U_X; -U_Y; U_Z]/T_THROTTLE_OUT;   
%     T_ROLL_OUT      = asin(Urot(2));
%     T_PITCH_OUT     = asin((Urot(1))/(-cos(T_ROLL_OUT)));    
% end

if(AUTO_FLIGHT)
    T_THROTTLE_OUT  = U_Z;
%     T_PITCH_OUT     = U_X/(-9.81);   
    
    T_ROLL_OUT      = U_Y/(9.81);
    T_PITCH_OUT     = T_PITCH_IN;   
    
%         Urot            = Rz*[-U_X; -U_Y; U_Z]/(-9.81);   
%     T_ROLL_OUT      = Urot(2);
%     T_PITCH_OUT     = Urot(1); 
       
end

%% Saturate output
if( abs(T_PITCH_OUT) > (pi/4) )
    T_PITCH_OUT = sign(T_PITCH_OUT)*(pi/4);
end

if( abs(T_ROLL_OUT) > (pi/4) )
    T_ROLL_OUT = sign(T_ROLL_OUT)*(pi/4);
end

== matlab function PX4_Run_Mode_R2016b/SENSOR_FILTER/SensorData2States/Translational State Estimation/MATLAB Function2 ==
  data: u input; Xhat output; z input; A parameter; B parameter; C_1 parameter; Q parameter; R_1 parameter; I parameter
function Xhat = KalmanFilter(u,z, A, B, C_1, Q, R_1, I)

%% Inputs
%   1   Latitude
%   2   Longitude
%   3   Altitude
%   4   Sonar

persistent Xhat_Old
if(isempty(Xhat_Old))
    Xhat_Old = single(zeros(6,1));
end

persistent P_Old
if(isempty(P_Old))
    P_Old = Q;
end

%% Initiate
Xhat = Xhat_Old;
P = P_Old;

%% Predict
Xhat = A * Xhat + B * u;
P = A * P * A' + Q;

%% Calculate gain
K = P * C_1' * inv(C_1 * P * C_1' + R_1);

%% Update
Xhat = Xhat + K * (z - C_1 * Xhat);
P = (I - K * C_1) * P;

%% Save Values for next iteration
P_Old = P;
Xhat_Old = Xhat;

== matlab function PX4_Run_Mode_R2016b/SENSOR_FILTER/Fixed Bias removal and scaling/Parameter Bus Creation/Madgewick Filter/Initial Madgewick ==
  data: y output; app parameter; Kapp parameter; thg parameter; m0 parameter; Dip0 parameter; thdip parameter; Beta parameter
function y = Initialize_Madgewick(app, Kapp, thg, m0, Dip0, thdip, Beta)

% app     = Maximum expected acceleration during stationary state (peak - peak)
% Kapp    = Stationary state detection accelerometer detection
% thg     = Maximum expected gyroscope during stationary state (bound)
% m0      = Expected Magnetometer magnitude
% Dip0    = Expected Dip angle under undisturbed operation
% thdip   = Scaling dip error
% Beta    = Gradient Descent Step size

y = [app; Kapp; thg; m0; Dip0; thdip; Beta];

== matlab function PX4_Run_Mode_R2016b/SENSOR_FILTER/Fixed Bias removal and scaling/Parameter Bus Creation/Kalman Filter/Initialize Kalman Filter ==
  data: Amat output; A parameter; B parameter; C parameter; D parameter; Q parameter; R parameter; pn parameter; mn parameter; Bmat output; Cmat output; Dmat output; Qmat output; Rmat output; pnvec output; mnvec output
function [Amat, Bmat, Cmat, Dmat, Qmat, Rmat, pnvec, mnvec] = Initialize_Kalman_Filter(A, B, C, D, Q, R, pn, mn)

% pn = [3, 1] Process noise Magnitude
% mn = [4, 1] Measurement noise Magnitude
% 
% A = [6, 6] State transition matrix
% B = [6, 3] Control input matrix
% C = [4, 6] Measurement matrix
% D = [4, 3] Feedthrough matrix
% 
% Q = [6, 6] Convert the process noise (stdv) into covariance matrix
% R = [4, 4] Convert the measurement noise (stdv) into covariance matrix

Amat = reshape(A,[36,1]);
Bmat = reshape(B,[18,1]);
Cmat = reshape(C,[24,1]);
Dmat = reshape(D,[12,1]);
Qmat = reshape(Q,[36,1]);
Rmat = reshape(R,[16,1]);

pnvec = pn;
mnvec = mn;
